simulink model "week3_prob2"  (R2020b)
settings: Solver=FixedStepDiscrete  StartTime=0.0  StopTime=inf  FixedStep=.1  RelTol=1e-3  EnableMultiTasking=on
libraries: simulink_extras x1
settings Model: Creator=The MathWorks, Inc.  LastModifiedBy=Lakshmi
settings DataIOCC: LimitDataPoints=on  SaveFormat=Array  ReturnWorkspaceOutputs=off
settings OptimizationCC: ExpressionDepthLimit=2147483647  InitFltsAndDblsToZero=on  EfficientMapNaN2IntZero=off  LifeSpan=inf
settings DebuggingCC: SaveWithParameterizedLinksMsg=none  UnderspecifiedInitializationDetection=Classic  MergeDetectMultiDrivingBlocksExec=none  SignalResolutionControl=TryResolveAllWithWarning  SolverPrmCheckMsg=warning  MultiTaskDSMMsg=warning  MultiTaskCondExecSysMsg=none  FcnCallInpInsideContextMsg=warning  StateNameClashWarn=warning  SFUnexpectedBacktrackingDiag=warning  SFNoUnconditionalDefaultTransitionDiag=warning  SFExecutionAtInitializationDiag=none  ArithmeticOperatorsInVariantConditions=warning
settings HardwareCC: ProdBitPerPointer=32  ProdBitPerSizeT=32  ProdBitPerPtrDiffT=32  ProdLargestAtomicFloat=None  ProdIntDivRoundTo=Undefined  ProdEndianess=Unspecified  ProdWordSize=32  ProdHWDeviceType=32-bit Generic
settings ModelReferenceCC: PropagateSignalLabelsOutOfModel=off
settings SFSimCC: SimUseLocalCustomCode=off  SimParseCustomCode=off  CustomCodeUndefinedFunction=UseInterfaceOnly
settings RTWCC: RTWUseLocalCustomCode=off
settings CodeAppCC: StateflowObjectComments=on
settings GRTTargetCC: TargetFcnLib=ansi_tfl_tmw.mat  TargetLangStandard=C89/C90 (ANSI)  CombineOutputUpdateFcns=off  GRTInterface=on
settings ConfigComp: CovMetricSettings=dw  CovSaveCumulativeToWorkspaceVar=on  CovSaveSingleToWorkspaceVar=on  CovExternalEMLEnable=off  CovSFcnEnable=off

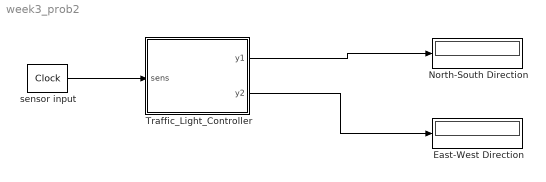
== system week3_prob2 ==
  East-West Direction : Display
  North-South Direction : Display
  Traffic_Light_Controller : Stateflow chart  TreatAsAtomicUnit=on
  sensor input : simulink_extras/Flip Flops/Clock  period=5
  wires:
  Traffic_Light_Controller/2(y2) -> East-West Direction/1
  Traffic_Light_Controller/1(y1) -> North-South Direction/1
  sensor input/1 -> Traffic_Light_Controller/1(sens)

== stateflow chart week3_prob2/Traffic_Light_Controller ==
  settings: stateMachineType=MOORE_MACHINE  executeAtInitialization=1  initializeOutput=1
  state Stop
    y1 = Red;
    y2 = Green;
  state StopForTraffic
    y1 = Red;
    y2 = Green;
  state StopToGo
    y1 = Red;
    y2 = Yellow;
  state GoToStop
    y1 = Yellow;
    y2 = Red;
  state Go
    y1 = Green;
    y2 = Red;
  (default) -> Stop
  StopForTraffic -> StopToGo : [sens]
  Stop -> StopForTraffic : after(20,tick)
  GoToStop -> Stop : after (3,tick)
  StopToGo -> Go : after(3,tick)
  Go -> GoToStop : after(10,tick)
  data: sens input double; y1 output double; y2 output double; Green constant double =3; Yellow constant double =2; Red constant double =1
